simulink model "Control_v6_LQR_2020b_for_Monte_carlo"  (R2020b)
settings: Solver=FixedStepAuto  StartTime=0.0  StopTime=t_sim  FixedStep=TimeStep  RelTol=1e-3
values from neighbouring files (symbols this model uses):
  K = [mean(Kq1)  0  0  mean(Kw1)  0  0 ... (first row only)    [LQR_Compute_feedback_gain_matrix.m]    (also in LQR_Monte_Carlo_initial_conditions.m = [0.00053417  0  0  0.0070506  0  0; Main_LQR_Monte_Carlo_Simulations.m = [0.00053417  0  0  0.0070506  0  0)
  sat_inertia = [I_xx I_xy I_xz ... (first row only)    [Main_LQR_Monte_Carlo_Simulations.m]
  Use_IGRF = 1    [LQR_Monte_Carlo_initial_conditions.m]    (also in Main_LQR_Monte_Carlo_Simulations.m)
undefined symbols (not defined in the file or in its folder): att, date, deg, DiscIntNeverNeededParam, IonSataero, km, MODE_SEQUENCE, orbit, rad, RW_failure_matrix, s, sat
libraries: vrlib x23, aerolibutil x15, dspmathops x15, aerolibconvert2 x14, sharedtransform x13, simulink x4, simulink_extras x2, aerolibatmos2 x1, DipoleModel x1, aerolibobsolete x1, sharedutil x1, aerolibcelestial x1
(part 1 of 3)
settings Model: EnablePacing=on  PacingRate=1000  Creator=colpari  LastModifiedBy=shinok.kang
settings SolverCC: ExtrapolationOrder=3
settings OptimizationCC: DefaultParameterBehavior=Inlined  UseDivisionForNetSlopeComputation=on  GainParamInheritBuiltInType=on  UseFloatMulNetSlope=on  InlineInvariantSignals=on  EfficientFloat2IntCast=on  LifeSpan=1
settings HardwareCC: ProdLongLongMode=on
settings SFSimCC: MATLABDynamicMemAlloc=off
settings RTWCC: GenerateReport=on  LaunchReport=on
settings CodeAppCC: ForceParamTrailComments=on
settings GRTTargetCC: CombineSignalStateStructs=on  MatFileLogging=off  SupportVariableSizeSignals=on

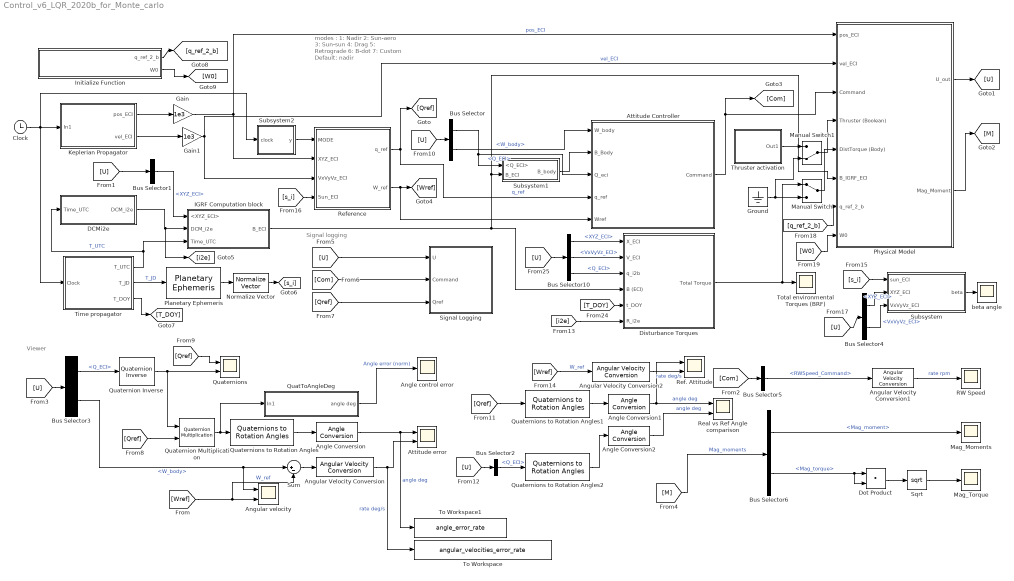
== system Control_v6_LQR_2020b_for_Monte_carlo ==
  note: Viewer
  note: Signal logging
  note: modes :
      | 1: Nadir
      | 2: Sun-aero
      | 3: Sun-sun
      | 4: Drag
      | 5: Retrograde
      | 6: B-dot
      | 7: Custom
      | Default: nadir
  Angle Conversion : aerolibconvert2/Angle Conversion  IU=rad  OU=deg
  Angle Conversion1 : aerolibconvert2/Angle Conversion  IU=rad  OU=deg
  Angle Conversion2 : aerolibconvert2/Angle Conversion  IU=rad  OU=deg
  Angle control error : Scope
  Angular Velocity Conversion : aerolibconvert2/Angular Velocity Conversion  IU=rad/s  OU=deg/s
  Angular Velocity Conversion1 : aerolibconvert2/Angular Velocity Conversion  IU=rad/s  OU=rpm
  Angular Velocity Conversion2 : aerolibconvert2/Angular Velocity Conversion  IU=rad/s  OU=deg/s
  Angular velocity : Scope  NumInputPorts=2
  Attitude Controller : Subsystem  TreatAsAtomicUnit=on
  Attitude error : Scope  NumInputPorts=2
  Bus Selector : BusSelector  OutputSignals=Q_ECI,W_body
  Bus Selector1 : BusSelector  OutputSignals=XYZ_ECI
  Bus Selector10 : BusSelector  OutputSignals=XYZ_ECI,VxVyVz_ECI,Q_ECI
  Bus Selector2 : BusSelector  OutputSignals=Q_ECI
  Bus Selector3 : BusSelector  OutputSignals=Q_ECI,W_body
  Bus Selector4 : BusSelector  OutputSignals=XYZ_ECI,VxVyVz_ECI
  Bus Selector5 : BusSelector  OutputSignals=RWSpeed_Command
  Bus Selector6 : BusSelector  OutputSignals=Mag_moment,Mag_torque
  Clock : Clock
  DCMi2e : Subsystem  TreatAsAtomicUnit=on  SystemSampleTime=1
  Disturbance Torques : Subsystem
  Dot Product : DotProduct  InputSameDT=on  OutDataTypeStr=Inherit: Inherit via internal rule
  Gain : Gain  Gain=1e3
  Gain1 : Gain  Gain=1e3
  Ground : Ground
  IGRF Computation block : Subsystem
  Initialize Function : Subsystem  TreatAsAtomicUnit=on
  Keplerian Propagator : Subsystem
  Mag_Moments : Scope
  Mag_Torque : Scope
  Manual Switch : ManualSwitch
  Manual Switch1 : ManualSwitch  CurrentSetting=0
  Normalize Vector : vrlib/Utilities/Normalize Vector  maxzero=0
  Physical Model : Subsystem
      settings: MinAlgLoopOccurrences=on
  Planetary Ephemeris : aerolibcelestial/Planetary Ephemeris  kmflag=km,km/s  epochflag=Julian date  de=DE405  nCenter=Earth  nTarget=Sun  errorflag=Error  velflag=off
      settings: SourceProductBaseCode=AE
  QuatToAngleDeg : Subsystem
  Quaternion Inverse : aerolibutil/Quaternion Inverse
  Quaternion Multiplication : aerolibutil/Quaternion Multiplication
  Quaternions : Scope  NumInputPorts=2
  Quaternions to Rotation Angles : sharedtransform/Quaternions to Rotation Angles  rotationOrder=ZYX  aMode=aMode
      settings: SourceProductBaseCode=AE,PW,DR,MT,UV,VE
  Quaternions to Rotation Angles1 : sharedtransform/Quaternions to Rotation Angles  rotationOrder=ZYX  aMode=aMode
      settings: SourceProductBaseCode=AE,PW,DR,MT,UV,VE
  Quaternions to Rotation Angles2 : sharedtransform/Quaternions to Rotation Angles  rotationOrder=ZYX  aMode=aMode
      settings: SourceProductBaseCode=AE,PW,DR,MT,UV,VE
  RW Speed : Scope
  Real vs Ref Angle comparison : Scope  NumInputPorts=2
  Ref. Attitude : Scope  NumInputPorts=2
  Reference : Subsystem  TreatAsAtomicUnit=on
  Signal Logging : Subsystem
  Sqrt : Sqrt  SaturateOnIntegerOverflow=on
  Subsystem : Subsystem
  Subsystem1 : Subsystem
  Subsystem2 : Subsystem
  Sum : Sum  Inputs=|+-
  Thruster activation : Subsystem
  Time propagator : Subsystem
  To Workspace : ToWorkspace  VariableName=angular_velocities_error_rate  SaveFormat=Timeseries  SampleTime=-1
  To Workspace1 : ToWorkspace  VariableName=angle_error_rate  SaveFormat=Timeseries  SampleTime=-1
  Total environmental Torques (BRF) : Scope
  beta angle : Scope
  wires:
  Clock/1 -> Subsystem2/1(clock), Keplerian Propagator/1(In1), Time propagator/1(Clock)
  Keplerian Propagator/1(pos_ECI) -> Gain/1
  Keplerian Propagator/2(vel_ECI) -> Gain1/1
  Planetary Ephemeris/1 -> Normalize Vector/1
  Time propagator/2(T_JD) -> Planetary Ephemeris/1  "T_JD"
  Reference/1(q_ref) -> [Qref], Attitude Controller/4(q_ref)  "q_ref"
  Physical Model/1(U_out) -> [U]
  Time propagator/1(T_UTC) -> DCMi2e/1(Time_UTC), IGRF Computation block/3("Time_UTC ")  "T_UTC"
  Gain/1 -> Reference/2(XYZ_ECI), Physical Model/1(pos_ECI)  "pos_ECI"
  Gain1/1 -> Reference/3(VxVyVz_ECI), Physical Model/2(vel_ECI)  "vel_ECI"
  Attitude Controller/1(Command) -> Physical Model/3(Command), [Com]
  IGRF Computation block/1(B_ECI) -> Physical Model/6(B_IGRF_ECI), Subsystem1/2(B_ECI), Disturbance Torques/4(B (ECI))
  [U] -> Bus Selector/1
  Bus Selector/1 -> Subsystem1/1(<Q_ECI>), Attitude Controller/3(Q_eci)  "<Q_ECI>"
  Bus Selector/2 -> Attitude Controller/1(W_body)  "<W_body>"
  [U] -> Bus Selector1/1
  Bus Selector1/1 -> IGRF Computation block/1(<XYZ_ECI>)  "<XYZ_ECI>"
  [Qref] -> Signal Logging/3(Qref)
  Quaternions to Rotation Angles/1 -> Angle Conversion/1
  Bus Selector6/2 -> Dot Product/2, Dot Product/1  "<Mag_torque>"
  Bus Selector6/1 -> Mag_Moments/1  "<Mag_moment>"
  Dot Product/1 -> Sqrt/1
  Bus Selector3/1 -> Quaternion Inverse/1  "<Q_ECI>"
  Sqrt/1 -> Mag_Torque/1
  Bus Selector5/1 -> Angular Velocity Conversion1/1  "<RWSpeed_Command>"
  [Com] -> Signal Logging/2(Command)
  [Com] -> Bus Selector5/1
  Bus Selector3/2 -> Sum/1, Angular velocity/1  "<W_body>"
  [U] -> Bus Selector3/1
  Quaternion Inverse/1 -> Quaternion Multiplication/1, Quaternions/2
  [M] -> Bus Selector6/1  "Mag_moments"
  Angular Velocity Conversion/1 -> To Workspace/1, Attitude error/2  "rate deg/s"
  Quaternion Multiplication/1 -> QuatToAngleDeg/1(In1), Quaternions to Rotation Angles/1
  [U] -> Signal Logging/1(U)
  Angle Conversion/1 -> To Workspace1/1, Attitude error/1  "angle deg"
  Angular Velocity Conversion1/1 -> RW Speed/1  "rate rpm"
  Physical Model/2(Mag_Moment) -> [M]
  Subsystem1/1(B_body) -> Attitude Controller/2(B_Body)
  QuatToAngleDeg/1(angle deg) -> Angle control error/1  "Angle error (norm)"
  Reference/2(W_ref) -> Attitude Controller/5(Wref), [Wref]
  [Wref] -> Sum/2, Angular velocity/2  "W_ref"
  Sum/1 -> Angular Velocity Conversion/1
  Angle Conversion1/1 -> Ref. Attitude/1, Real vs Ref Angle comparison/1  "angle deg"
  Quaternions to Rotation Angles1/1 -> Angle Conversion1/1
  Thruster activation/1(Out1) -> Manual Switch1/1
  [U] -> Bus Selector10/1
  [T_DOY] -> Disturbance Torques/5(t_DOY)
  Bus Selector10/3 -> Disturbance Torques/3(q_i2b)  "<Q_ECI>"
  Time propagator/3(T_DOY) -> [T_DOY]
  Manual Switch/1 -> Physical Model/5(DistTorque (Body))
  Ground/1 -> Manual Switch/2, Manual Switch1/2
  Bus Selector2/1 -> Quaternions to Rotation Angles2/1  "<Q_ECI>"
  Quaternions to Rotation Angles2/1 -> Angle Conversion2/1
  Angle Conversion2/1 -> Real vs Ref Angle comparison/2  "angle deg"
  [U] -> Bus Selector2/1
  [Wref] -> Angular Velocity Conversion2/1  "W_ref"
  Angular Velocity Conversion2/1 -> Ref. Attitude/2  "rate deg/s"
  DCMi2e/1(DCM_i2e) -> [i2e], IGRF Computation block/2("DCM_i2e ")
  [i2e] -> Disturbance Torques/6(R_i2e)
  Bus Selector10/1 -> Disturbance Torques/1(X_ECI)  "<XYZ_ECI>"
  Bus Selector10/2 -> Disturbance Torques/2(V_ECI)  "<VxVyVz_ECI>"
  Manual Switch1/1 -> Physical Model/4(Thruster (Boolean))
  Subsystem2/1(y) -> Reference/1(MODE)
  [s_i] -> Subsystem/1(sun_ECI)
  Subsystem/1(beta) -> beta angle/1
  Normalize Vector/1 -> [s_i]
  [s_i] -> Reference/4(Sun_ECI)
  [U] -> Bus Selector4/1
  Bus Selector4/1 -> Subsystem/2(XYZ_ECI)  "<XYZ_ECI>"
  Bus Selector4/2 -> Subsystem/3(VxVyVz_ECI)  "<VxVyVz_ECI>"
  Disturbance Torques/1("Total Torque ") -> Total environmental Torques (BRF)/1, Manual Switch/1
  [Qref] -> Quaternions to Rotation Angles1/1
  [Qref] -> Quaternions/1
  [Qref] -> Quaternion Multiplication/2
  Initialize Function/1(q_ref_2_b) -> [q_ref_2_b]
  [q_ref_2_b] -> Physical Model/7(q_ref_2_b)
  [W0] -> Physical Model/8(W0)
  Initialize Function/2(W0) -> [W0]

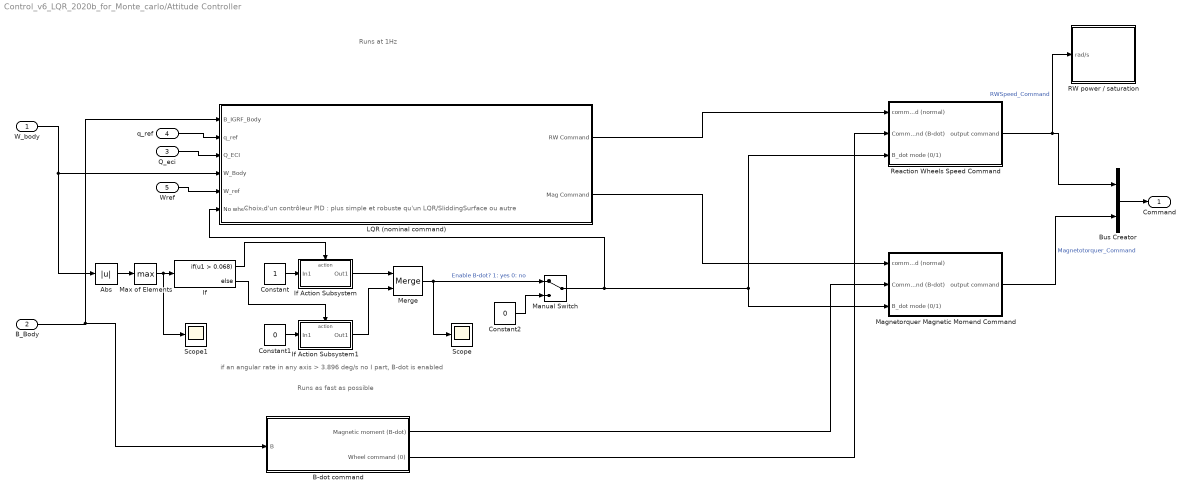
== system Control_v6_LQR_2020b_for_Monte_carlo/Attitude Controller ==
  note: Choix d'un contrôleur PID : plus simple et robuste qu'un LQR/SliddingSurface ou autre
  note: Runs as fast as possible
  note: Runs at 1Hz
  note: if an angular rate in any axis > 3.896 deg/s no I part, B-dot is enabled
  W_body : Inport
  B_Body : Inport  Port=2
  Q_eci : Inport  Port=3
  q_ref : Inport  Port=4
  Wref : Inport  Port=5
  Abs : Abs
  B-dot command : Subsystem  TreatAsAtomicUnit=on
  Bus Creator : BusCreator  Inputs=2
  Constant : Constant
  Constant1 : Constant  Value=0
  Constant2 : Constant  Value=0
  If : If  IfExpression=u1 > 0.068
  If Action Subsystem : Subsystem  TreatAsAtomicUnit=on
  If Action Subsystem1 : Subsystem  TreatAsAtomicUnit=on
  LQR (nominal command) : Subsystem  TreatAsAtomicUnit=on
  Magnetorquer Magnetic Momend Command : Subsystem
  Manual Switch : ManualSwitch
  Max of Elements : MinMax  Function=max
  Merge : Merge
  RW power / saturation : Subsystem
  Reaction Wheels Speed Command : Subsystem
  Scope : Scope
  Scope1 : Scope
  Command : Outport  VectorParamsAs1DForOutWhenUnconnected=off
  wires:
  B_Body/1 -> B-dot command/1(B), LQR (nominal command)/1(B_IGRF_Body)
  Magnetorquer Magnetic Momend Command/1(output command) -> Bus Creator/2  "Magnetotorquer_Command"
  Reaction Wheels Speed Command/1(output command) -> RW power / saturation/1(rad/s), Bus Creator/1  "RWSpeed_Command"
  B-dot command/2(Wheel command (0)) -> Reaction Wheels Speed Command/2(Command (B-dot))
  B-dot command/1(Magnetic moment (B-dot)) -> Magnetorquer Magnetic Momend Command/2(Command (B-dot))
  LQR (nominal command)/1(RW Command) -> Reaction Wheels Speed Command/1(" command (normal)")
  LQR (nominal command)/2(Mag Command) -> Magnetorquer Magnetic Momend Command/1(" command (normal)")
  Bus Creator/1 -> Command/1
  Abs/1 -> Max of Elements/1
  If/1 -> If Action Subsystem/Action
  If Action Subsystem1/1(Out1) -> Merge/2
  Max of Elements/1 -> Scope1/1, If/1
  If/2 -> If Action Subsystem1/Action
  If Action Subsystem/1(Out1) -> Merge/1
  Constant/1 -> If Action Subsystem/1(In1)
  Merge/1 -> Manual Switch/1, Scope/1  "Enable B-dot? 1: yes 0: no"
  Constant1/1 -> If Action Subsystem1/1(In1)
  W_body/1 -> Abs/1, LQR (nominal command)/4(W_Body)
  Wref/1 -> LQR (nominal command)/5(W_ref)
  q_ref/1 -> LQR (nominal command)/2(q_ref)
  Q_eci/1 -> LQR (nominal command)/3(Q_ECI)
  Constant2/1 -> Manual Switch/2
  Manual Switch/1 -> LQR (nominal command)/6(No wheels use), Reaction Wheels Speed Command/3(B_dot mode (0/1)), Magnetorquer Magnetic Momend Command/3(B_dot mode (0/1))

== system Control_v6_LQR_2020b_for_Monte_carlo/DCMi2e ==
  note: Slower subsytem because it's too slow
  Time_UTC : Inport
  ECI to ECEF : MATLABFcn  MATLABFcn=eci2ecef  OutputDimensions=[3;3]  Output1D=off
  DCM_i2e : Outport
  wires:
  ECI to ECEF/1 -> DCM_i2e/1
  Time_UTC/1 -> ECI to ECEF/1

== system Control_v6_LQR_2020b_for_Monte_carlo/Disturbance Torques ==
  X_ECI : Inport
  V_ECI : Inport  Port=2
  q_i2b : Inport  Port=3
  B (ECI) : Inport  Port=4
  t_DOY : Inport  Port=5
  R_i2e : Inport  Port=6
  3 dist torques : Scope  NumInputPorts=3
  Add1 : Sum  Inputs=+++
  Aerodynamic Model : Subsystem
  Gravity Gradient Model : Subsystem
  Ground : Ground
  Ground1 : Ground
  Ground2 : Ground
  Magnetic Torque Model : Subsystem
  Manual Switch : ManualSwitch
  Manual Switch1 : ManualSwitch
  Manual Switch2 : ManualSwitch
  Quaternions to Direction Cosine Matrix : sharedtransform/Quaternions to  Direction Cosine Matrix  aMode=aMode
      settings: SourceProductBaseCode=AE,PW,DR,MT,UV,VE
  To Workspace : ToWorkspace  VariableName=aerotorque  SaveFormat=Timeseries  SampleTime=-1
  Total Torque : Scope
  "Total Torque " : Outport
  wires:
  Add1/1 -> Total Torque/1, "Total Torque "/1
  V_ECI/1 -> Aerodynamic Model/1(Velocity  (V) [m/s])
  X_ECI/1 -> Aerodynamic Model/2(Position (X) [m]), Gravity Gradient Model/1("Position (X) [m] ")
  Manual Switch/1 -> 3 dist torques/1, Add1/1  "Aero Torque"
  Manual Switch2/1 -> Add1/3, 3 dist torques/3  "GG Torque"
  B (ECI)/1 -> Magnetic Torque Model/1(B (ECI))
  Manual Switch1/1 -> Add1/2, 3 dist torques/2  "Magnetic Torque"
  q_i2b/1 -> Quaternions to Direction Cosine Matrix/1
  Quaternions to Direction Cosine Matrix/1 -> Gravity Gradient Model/2(Attitude (DCMi2b)), Magnetic Torque Model/2(Attitude (DCMi2b)), Aerodynamic Model/3(Attitude (DCM_i2b))  "i2b"
  R_i2e/1 -> Aerodynamic Model/5(DCM_i2e)
  t_DOY/1 -> Aerodynamic Model/4(DOY)
  Ground/1 -> Manual Switch/2
  Aerodynamic Model/1(Aero. Torque [N.m]) -> To Workspace/1, Manual Switch/1  "Aero Torque"
  Magnetic Torque Model/1(MagneticTorque (N.m)) -> Manual Switch1/1  "Magnetic Torque"
  Ground1/1 -> Manual Switch1/2
  Ground2/1 -> Manual Switch2/2
  Gravity Gradient Model/1(Gravity Gradient [N.m]) -> Manual Switch2/1  "GG Torque"

== system Control_v6_LQR_2020b_for_Monte_carlo/IGRF Computation block ==
  <XYZ_ECI> : Inport
  "DCM_i2e " : Inport  Port=2
  "Time_UTC " : Inport  Port=3
  Bus Creator : BusCreator  Inputs=5
  Bus Selector4 : BusSelector  OutputSignals=XYZ_ECI
  Constant : Constant  Value=[0.4;0.4;0.4]
  Cross Product : vrlib/Utilities/Cross Product
  Demux : Demux  Outputs=2
  ECI To LLA : MATLAB Function  TreatAsAtomicUnit=on
  MATLAB Function : MATLAB Function  TreatAsAtomicUnit=on
  Mux : Mux  Inputs=3
  Obtain B_ECI : Subsystem
  Product : Product  Multiplication=Matrix(*)
  Reshape : Reshape  OutputDimensionality=Row vector (2-D)
  Scope : Scope
  Terminator : Terminator
  To Workspace : ToWorkspace  VariableName=B_ECI  SaveFormat=Timeseries  SampleTime=-1
  B_ECI : Outport  VectorParamsAs1DForOutWhenUnconnected=off
  wires:
  ECI To LLA/3(long) -> Bus Creator/3
  ECI To LLA/2(lat) -> Bus Creator/2
  ECI To LLA/1(h) -> Bus Creator/1
  Demux/1 -> Bus Creator/4  "time_UTC"
  Demux/2 -> Terminator/1
  "DCM_i2e "/1 -> Product/2, Bus Creator/5  "DCM_i2e"
  <XYZ_ECI>/1 -> Bus Selector4/1
  Reshape/1 -> Product/1
  Product/1 -> ECI To LLA/1(X_ECEF)
  Bus Selector4/1 -> Reshape/1  "<XYZ_ECI>"
  Bus Creator/1 -> Obtain B_ECI/1(In1)
  Obtain B_ECI/1(u) -> Cross Product/2, MATLAB Function/1(u), Mux/1, To Workspace/1, B_ECI/1
  "Time_UTC "/1 -> Demux/1
  Mux/1 -> Scope/1
  MATLAB Function/1(y) -> Mux/2
  Constant/1 -> Cross Product/1
  Cross Product/1 -> Mux/3

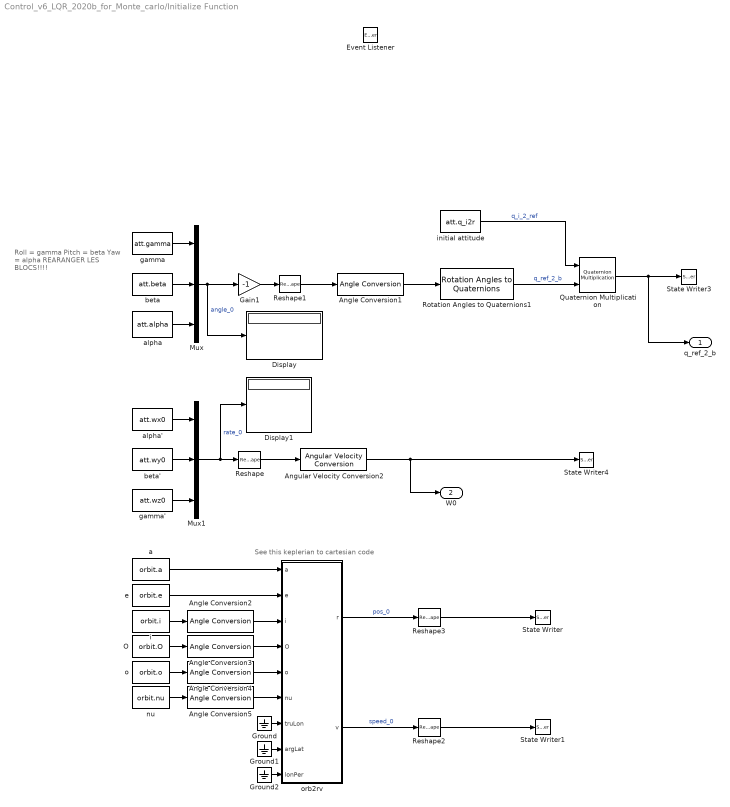
== system Control_v6_LQR_2020b_for_Monte_carlo/Initialize Function ==
  note: Roll = gamma
      | Pitch = beta
      | Yaw = alpha
      | REARANGER LES BLOCS!!!!
  note: See this keplerian to cartesian code
  Angle Conversion{1..5} (5 alike) : aerolibconvert2/Angle Conversion  IU=deg  OU=rad
  Angular Velocity Conversion2 : aerolibconvert2/Angular Velocity Conversion  IU=deg/s  OU=rad/s
  Display : Display
  Display1 : Display
  Event Listener : EventListener  DisableCoverage=on  EventName=reset
  Gain1 : Gain  Gain=-1
  Ground : Ground
  Ground1 : Ground
  Ground2 : Ground
  Mux : Mux  Inputs=3
  Mux1 : Mux  Inputs=3
  O : Constant  Value=orbit.O
  Quaternion Multiplication : aerolibutil/Quaternion Multiplication
  Reshape{,1..3} (4 alike) : Reshape  OutputDimensionality=Column vector (2-D)
  Rotation Angles to Quaternions1 : sharedtransform/Rotation Angles to Quaternions  rotationOrder=XYZ  aMode=aMode
      settings: SourceProductBaseCode=AE,PW,DR,MT,UV,VE
  State Writer : StateWriter  StateOwnerBlock=../../Keplerian Propagator/Integrator
  State Writer1 : StateWriter  StateOwnerBlock=../../Keplerian Propagator/Integrator1
  State Writer3 : StateWriter  StateOwnerBlock=../../Physical Model/6DOF in ECI frame/Compute Q_ECI/Integrator_quat
  State Writer4 : StateWriter  StateOwnerBlock=../../Physical Model/6DOF in ECI frame/Integrator_rate
  a : Constant  Value=orbit.a
  alpha : Constant  Value=att.alpha
  alpha' : Constant  Value=att.wx0
  beta : Constant  Value=att.beta
  beta' : Constant  Value=att.wy0
  e : Constant  Value=orbit.e
  gamma : Constant  Value=att.gamma
  gamma' : Constant  Value=att.wz0
  i : Constant  Value=orbit.i
  initial attitude : Constant  Value=att.q_i2r
  nu : Constant  Value=orbit.nu
  o : Constant  Value=orbit.o
  orb2rv : MATLAB Function  TreatAsAtomicUnit=on
  q_ref_2_b : Outport
  W0 : Outport  Port=2
  wires:
  Angular Velocity Conversion2/1 -> W0/1, State Writer4/1
  Mux1/1 -> Display1/1, Reshape/1  "rate_0"
  Reshape/1 -> Angular Velocity Conversion2/1
  alpha'/1 -> Mux1/1
  gamma'/1 -> Mux1/3
  beta'/1 -> Mux1/2
  Reshape3/1 -> State Writer/1
  i/1 -> Angle Conversion2/1
  Ground/1 -> orb2rv/7(truLon)
  Angle Conversion2/1 -> orb2rv/3(i)
  nu/1 -> Angle Conversion5/1
  Ground2/1 -> orb2rv/9(lonPer)
  Angle Conversion3/1 -> orb2rv/4(O)
  Angle Conversion5/1 -> orb2rv/6(nu)
  Ground1/1 -> orb2rv/8(argLat)
  o/1 -> Angle Conversion4/1
  a/1 -> orb2rv/1(a)
  O/1 -> Angle Conversion3/1
  orb2rv/2(v) -> Reshape2/1  "speed_0"
  e/1 -> orb2rv/2(e)
  orb2rv/1(r) -> Reshape3/1  "pos_0"
  Angle Conversion4/1 -> orb2rv/5(o)
  Reshape2/1 -> State Writer1/1
  Reshape1/1 -> Angle Conversion1/1
  Angle Conversion1/1 -> Rotation Angles to Quaternions1/1
  beta/1 -> Mux/2
  alpha/1 -> Mux/3
  gamma/1 -> Mux/1
  Mux/1 -> Gain1/1, Display/1  "angle_0"
  initial attitude/1 -> Quaternion Multiplication/1  "q_i_2_ref"
  Rotation Angles to Quaternions1/1 -> Quaternion Multiplication/2  "q_ref_2_b"
  Quaternion Multiplication/1 -> q_ref_2_b/1, State Writer3/1
  Gain1/1 -> Reshape1/1

== system Control_v6_LQR_2020b_for_Monte_carlo/Keplerian Propagator ==
  In1 : Inport
  Constant : Constant  Value=[0;0;0]
  Demux : Demux  Outputs=2
  Integrator : Integrator
  Integrator1 : Integrator
  Mux : Mux  Inputs=2
  Mux1 : Mux  Inputs=2
  Reshape1 : Reshape  OutputDimensionality=Customize  OutputDimensions=[6,1]
  Reshape3 : Reshape  OutputDimensionality=Column vector (2-D)
  keplerian propagator : MATLABFcn  MATLABFcn=kep_propagator
  pos_ECI : Outport
  vel_ECI : Outport  Port=2
  wires:
  Demux/2 -> vel_ECI/1  "vel_ECI"
  Demux/1 -> pos_ECI/1  "pos_ECI"
  keplerian propagator/1 -> Demux/1
  Mux1/1 -> keplerian propagator/1
  In1/1 -> Mux1/2
  Mux/1 -> Reshape1/1
  Reshape1/1 -> Mux1/1
  Integrator1/1 -> Mux/2
  Constant/1 -> Reshape3/1
  Reshape3/1 -> Integrator1/1, Integrator/1
  Integrator/1 -> Mux/1

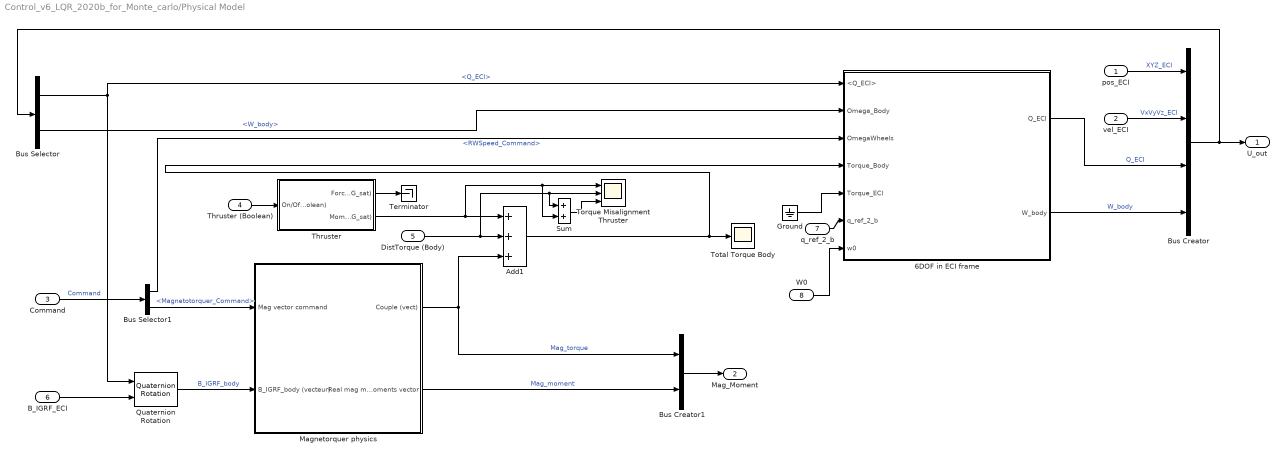
== system Control_v6_LQR_2020b_for_Monte_carlo/Physical Model ==
  pos_ECI : Inport
  vel_ECI : Inport  Port=2
  Command : Inport  Port=3
  Thruster (Boolean) : Inport  Port=4
  DistTorque (Body) : Inport  Port=5
  B_IGRF_ECI : Inport  Port=6
  q_ref_2_b : Inport  Port=7
  W0 : Inport  Port=8
  6DOF in ECI frame : Subsystem
  Add1 : Sum  Inputs=+++
  Bus Creator : BusCreator  Inputs=4
  Bus Creator1 : BusCreator  Inputs=2
  Bus Selector : BusSelector  OutputSignals=Q_ECI,W_body
  Bus Selector1 : BusSelector  OutputSignals=RWSpeed_Command,Magnetotorquer_Command
  Ground : Ground
  Magnetorquer physics : Subsystem
  Quaternion Rotation : aerolibutil/Quaternion Rotation
  Sum : Sum
  Terminator : Terminator
  Thruster : Subsystem
  Torque Misalignment Thruster : Scope  NumInputPorts=3
  Total Torque Body : Scope
  U_out : Outport  VectorParamsAs1DForOutWhenUnconnected=off
  Mag_Moment : Outport  Port=2  VectorParamsAs1DForOutWhenUnconnected=off
  wires:
  Thruster (Boolean)/1 -> Thruster/1(On/Off (Boolean))
  Bus Creator/1 -> U_out/1, Bus Selector/1
  Bus Selector/1 -> Quaternion Rotation/1, 6DOF in ECI frame/1(<Q_ECI>)  "<Q_ECI>"
  6DOF in ECI frame/1(Q_ECI) -> Bus Creator/3  "Q_ECI"
  Bus Selector1/2 -> Magnetorquer physics/1(Mag vector command)  "<Magnetotorquer_Command>"
  Thruster/2(Moment (G_sat)) -> Sum/2, Torque Misalignment Thruster/1, Add1/1
  Add1/1 -> Total Torque Body/1, 6DOF in ECI frame/4(Torque_Body)
  DistTorque (Body)/1 -> Sum/1, Torque Misalignment Thruster/2, Add1/2
  Bus Selector/2 -> 6DOF in ECI frame/2("Omega_Body ")  "<W_body>"
  B_IGRF_ECI/1 -> Quaternion Rotation/2
  Quaternion Rotation/1 -> Magnetorquer physics/2(B_IGRF_body (vecteur))  "B_IGRF_body"
  Magnetorquer physics/2(Real mag moments vector) -> Bus Creator1/2  "Mag_moment"
  Magnetorquer physics/1(Couple (vect)) -> Add1/3, Bus Creator1/1  "Mag_torque"
  6DOF in ECI frame/2(W_body) -> Bus Creator/4  "W_body"
  Command/1 -> Bus Selector1/1  "Command"
  Bus Selector1/1 -> 6DOF in ECI frame/3(OmegaWheels)  "<RWSpeed_Command>"
  Bus Creator1/1 -> Mag_Moment/1
  pos_ECI/1 -> Bus Creator/1  "XYZ_ECI"
  vel_ECI/1 -> Bus Creator/2  "VxVyVz_ECI"
  Thruster/1(Force (G_sat)) -> Terminator/1
  Ground/1 -> 6DOF in ECI frame/5(Torque_ECI)
  Sum/1 -> Torque Misalignment Thruster/3
  q_ref_2_b/1 -> 6DOF in ECI frame/6(q_ref_2_b)
  W0/1 -> 6DOF in ECI frame/7(w0)

== system Control_v6_LQR_2020b_for_Monte_carlo/QuatToAngleDeg ==
  In1 : Inport
  Abs : Abs
  Angle Conversion1 : aerolibconvert2/Angle Conversion  IU=rad  OU=deg
  Demux1 : Demux
  Quaternion to axis and angle conversion : MATLABFcn  MATLABFcn=quat2axisangle
  Terminator1 : Terminator
  Terminator2 : Terminator
  Terminator3 : Terminator
  angle deg : Outport  VectorParamsAs1DForOutWhenUnconnected=off
  wires:
  Demux1/2 -> Terminator2/1
  Demux1/4 -> Angle Conversion1/1
  In1/1 -> Quaternion to axis and angle conversion/1
  Demux1/1 -> Terminator1/1
  Demux1/3 -> Terminator3/1
  Quaternion to axis and angle conversion/1 -> Demux1/1
  Abs/1 -> angle deg/1
  Angle Conversion1/1 -> Abs/1  "angle deg"

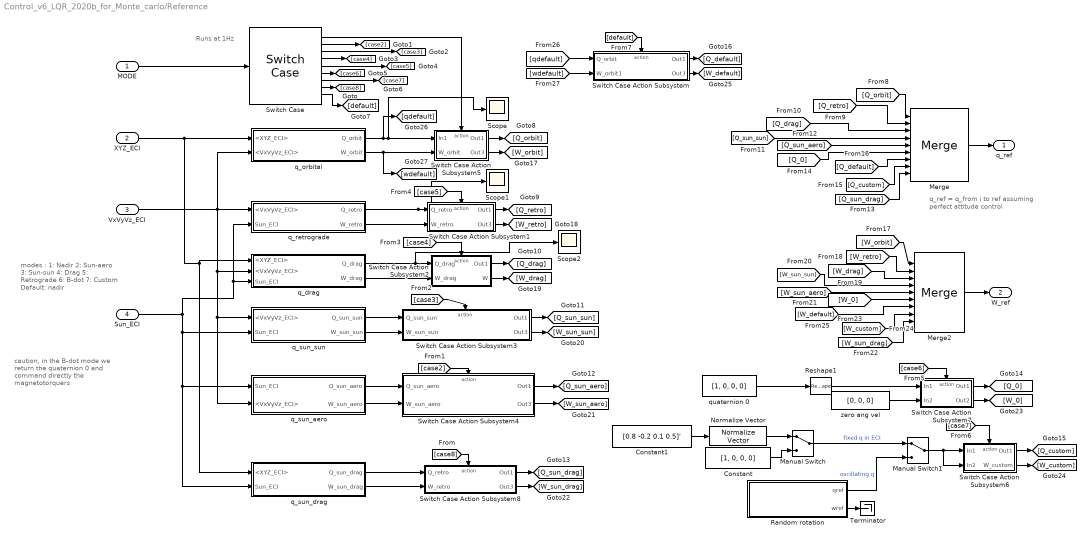
== system Control_v6_LQR_2020b_for_Monte_carlo/Reference ==
  note: caution, in the B-dot mode we return the quaternion 0 and command directly the magnetotorquers
  note: modes :
      | 1: Nadir
      | 2: Sun-aero
      | 3: Sun-sun
      | 4: Drag
      | 5: Retrograde
      | 6: B-dot
      | 7: Custom
      | Default: nadir
  note: q_ref  = q_from i to ref
      | assuming perfect attitude control
  note: Runs at 1Hz
  MODE : Inport  OutMin=1  OutMax=100  OutDataTypeStr=int8
  XYZ_ECI : Inport  Port=2
  VxVyVz_ECI : Inport  Port=3
  Sun_ECI : Inport  Port=4
  Constant : Constant  Value=[1, 0, 0, 0]
  Constant1 : Constant  Value=[0.8 -0.2 0.1 0.5]'
  Manual Switch : ManualSwitch
  Manual Switch1 : ManualSwitch
  Merge : Merge  Inputs=9
  Merge2 : Merge  Inputs=9
  Normalize Vector : vrlib/Utilities/Normalize Vector  maxzero=0
  Random rotation : Subsystem
  Reshape1 : Reshape  OutputDimensionality=Column vector (2-D)
  Scope : Scope
  Scope1 : Scope
  Scope2 : Scope
  Switch Case : SwitchCase  CaseConditions={1, 2, 3, 4, 5, 6, 7, 8}
  Switch Case Action Subsystem : Subsystem  TreatAsAtomicUnit=on
  Switch Case Action Subsystem1 : Subsystem  TreatAsAtomicUnit=on
  Switch Case Action Subsystem2 : Subsystem  TreatAsAtomicUnit=on
  Switch Case Action Subsystem3 : Subsystem  TreatAsAtomicUnit=on
  Switch Case Action Subsystem4 : Subsystem  TreatAsAtomicUnit=on
  Switch Case Action Subsystem5 : Subsystem  TreatAsAtomicUnit=on
  Switch Case Action Subsystem6 : Subsystem  TreatAsAtomicUnit=on
  Switch Case Action Subsystem7 : Subsystem  TreatAsAtomicUnit=on
  Switch Case Action Subsystem8 : Subsystem  TreatAsAtomicUnit=on
  Terminator : Terminator
  q_drag : Subsystem
  q_orbital : Subsystem
  q_retrograde : Subsystem
  q_sun_aero : Subsystem
  q_sun_drag : Subsystem
  q_sun_sun : Subsystem
  quaternion 0 : Constant  Value=[1, 0, 0, 0]
  zero ang vel : Constant  Value=[0, 0, 0]
  q_ref : Outport  VectorParamsAs1DForOutWhenUnconnected=off
  W_ref : Outport  Port=2
  wires:
  quaternion 0/1 -> Reshape1/1
  Reshape1/1 -> Switch Case Action Subsystem7/1(In1)
  Constant/1 -> Manual Switch/2
  Constant1/1 -> Normalize Vector/1
  Normalize Vector/1 -> Manual Switch/1
  zero ang vel/1 -> Switch Case Action Subsystem7/2(In2)
  Manual Switch/1 -> Manual Switch1/1  "fixed q in ECI"
  Random rotation/1(qref) -> Manual Switch1/2  "oscillating q"
  Manual Switch1/1 -> Switch Case Action Subsystem6/2(In2), Switch Case Action Subsystem6/1(In1)
  XYZ_ECI/1 -> q_sun_drag/1(<XYZ_ECI>), q_drag/1(<XYZ_ECI>), q_orbital/1(<XYZ_ECI>)
  [default] -> Switch Case Action Subsystem/Action
  Switch Case/7 -> [case7]
  Switch Case/4 -> [case4]
  Switch Case/5 -> [case5]
  [case3] -> Switch Case Action Subsystem3/Action
  [case5] -> Switch Case Action Subsystem1/Action
  Switch Case/3 -> [case3]
  Switch Case/2 -> [case2]
  q_drag/2(W_drag) -> Switch Case Action Subsystem2/2(W_drag)
  q_sun_drag/2(W_sun_drag) -> Switch Case Action Subsystem8/2(W_retro)
  q_sun_aero/2(W_sun_aero) -> Switch Case Action Subsystem4/2(W_sun_aero)
  Switch Case/1 -> Switch Case Action Subsystem5/Action
  [case8] -> Switch Case Action Subsystem8/Action
  Switch Case/8 -> [case8]
  q_drag/1(Q_drag) -> Scope2/1, Switch Case Action Subsystem2/1(Q_drag)
  Switch Case/9 -> [default]
  Sun_ECI/1 -> q_drag/3(Sun_ECI), q_retrograde/2(Sun_ECI), q_sun_drag/2(Sun_ECI), q_sun_aero/1(Sun_ECI), q_sun_sun/2(Sun_ECI)
  q_sun_sun/2(W_sun_sun) -> Switch Case Action Subsystem3/2(W_sun_sun)
  q_retrograde/2(W_retro) -> Switch Case Action Subsystem1/2(W_retro)
  q_sun_sun/1(Q_sun_sun) -> Switch Case Action Subsystem3/1(Q_sun_sun)
  q_sun_aero/1(Q_sun_aero) -> Switch Case Action Subsystem4/1(Q_sun_aero)
  q_sun_drag/1(Q_sun_drag) -> Switch Case Action Subsystem8/1(Q_retro)
  Merge2/1 -> W_ref/1
  [case2] -> Switch Case Action Subsystem4/Action
  [case4] -> Switch Case Action Subsystem2/Action
  q_orbital/1(Q_orbit) -> [qdefault], Switch Case Action Subsystem5/1(In1), Scope/1
  q_retrograde/1(Q_retro) -> Switch Case Action Subsystem1/1(Q_retro), Scope1/1
  q_orbital/2(W_orbit) -> [wdefault], Switch Case Action Subsystem5/2(W_orbit)
  Switch Case/6 -> [case6]
  VxVyVz_ECI/1 -> q_orbital/2(<VxVyVz_ECI>), q_retrograde/1(<VxVyVz_ECI>), q_sun_aero/2(<VxVyVz_ECI>), q_sun_sun/1(<VxVyVz_ECI>), q_drag/2(<VxVyVz_ECI>)
  Merge/1 -> q_ref/1
  MODE/1 -> Switch Case/1
  Random rotation/2(wref) -> Terminator/1
  [case6] -> Switch Case Action Subsystem7/Action
  [case7] -> Switch Case Action Subsystem6/Action
  Switch Case Action Subsystem5/1(Out1) -> [Q_orbit]
  [Q_orbit] -> Merge/1
  Switch Case Action Subsystem1/1(Out1) -> [Q_retro]
  [Q_retro] -> Merge/2
  Switch Case Action Subsystem2/1(Out1) -> [Q_drag]
  [Q_drag] -> Merge/3
  Switch Case Action Subsystem3/1(Out1) -> [Q_sun_sun]
  [Q_sun_sun] -> Merge/4
  Switch Case Action Subsystem4/1(Out1) -> [Q_sun_aero]
  [Q_sun_aero] -> Merge/5
  Switch Case Action Subsystem8/1(Out1) -> [Q_sun_drag]
  [Q_sun_drag] -> Merge/9
  Switch Case Action Subsystem7/1(Out1) -> [Q_0]
  [Q_0] -> Merge/6
  Switch Case Action Subsystem6/1(Out1) -> [Q_custom]
  [Q_custom] -> Merge/8
  Switch Case Action Subsystem/1(Out1) -> [Q_default]
  [Q_default] -> Merge/7
  Switch Case Action Subsystem5/2(Out3) -> [W_orbit]
  [W_orbit] -> Merge2/1
  Switch Case Action Subsystem1/2(Out3) -> [W_retro]
  [W_retro] -> Merge2/2
  Switch Case Action Subsystem2/2(W) -> [W_drag]
  [W_drag] -> Merge2/3
  Switch Case Action Subsystem3/2(Out3) -> [W_sun_sun]
  [W_sun_sun] -> Merge2/4
  Switch Case Action Subsystem4/2(Out3) -> [W_sun_aero]
  [W_sun_aero] -> Merge2/5
  Switch Case Action Subsystem8/2(Out3) -> [W_sun_drag]
  [W_sun_drag] -> Merge2/9
  Switch Case Action Subsystem7/2(Out2) -> [W_0]
  [W_0] -> Merge2/6
  Switch Case Action Subsystem6/2(W_custom) -> [W_custom]
  [W_custom] -> Merge2/8
  Switch Case Action Subsystem/2(Out3) -> [W_default]
  [W_default] -> Merge2/7
  [qdefault] -> Switch Case Action Subsystem/1(Q_orbit)
  [wdefault] -> Switch Case Action Subsystem/2(W_orbit1)

== system Control_v6_LQR_2020b_for_Monte_carlo/Signal Logging ==
  U : Inport
  Command : Inport  Port=2
  Qref : Inport  Port=3
  Bus Selector : BusSelector  OutputSignals=RWSpeed_Command,Magnetotorquer_Command
  Bus Selector4 : BusSelector  OutputSignals=XYZ_ECI,VxVyVz_ECI,Q_ECI,W_body
  Reshape : Reshape
  Reshape1 : Reshape
  Reshape2 : Reshape
  To Workspace : ToWorkspace  VariableName=sat_pos  SaveFormat=Timeseries  SampleTime=1
      settings: Save2DSignal=2-D array (concatenate along first dimension)
  To Workspace1 : ToWorkspace  VariableName=sat_speed  SaveFormat=Timeseries  SampleTime=1
      settings: Save2DSignal=2-D array (concatenate along first dimension)
  To Workspace2 : ToWorkspace  VariableName=sat_Q  SaveFormat=Timeseries  SampleTime=1
      settings: Save2DSignal=2-D array (concatenate along first dimension)
  To Workspace3 : ToWorkspace  VariableName=sat_omega  SaveFormat=Timeseries  SampleTime=1
      settings: Save2DSignal=2-D array (concatenate along first dimension)
  To Workspace4 : ToWorkspace  VariableName=RWSpeed_Command  SaveFormat=Timeseries  SampleTime=1
      settings: Save2DSignal=2-D array (concatenate along first dimension)
  To Workspace5 : ToWorkspace  VariableName=sat_Qc  SaveFormat=Timeseries  SampleTime=1
      settings: Save2DSignal=2-D array (concatenate along first dimension)
  To Workspace6 : ToWorkspace  VariableName=Mag_Command  SaveFormat=Timeseries  SampleTime=1
      settings: Save2DSignal=2-D array (concatenate along first dimension)
  wires:
  Bus Selector4/3 -> To Workspace2/1  "<Q_ECI>"
  Bus Selector4/4 -> To Workspace3/1  "<W_body>"
  U/1 -> Bus Selector4/1
  Bus Selector4/2 -> To Workspace1/1  "<VxVyVz_ECI>"
  Command/1 -> Bus Selector/1
  Bus Selector4/1 -> To Workspace/1  "<XYZ_ECI>"
  Qref/1 -> Reshape1/1
  Reshape/1 -> To Workspace4/1
  Reshape1/1 -> To Workspace5/1
  Bus Selector/1 -> Reshape/1  "<RWSpeed_Command>"
  Bus Selector/2 -> Reshape2/1  "<Magnetotorquer_Command>"
  Reshape2/1 -> To Workspace6/1

== system Control_v6_LQR_2020b_for_Monte_carlo/Subsystem ==
  sun_ECI : Inport
  XYZ_ECI : Inport  Port=2
  VxVyVz_ECI : Inport  Port=3
  Acos : Trigonometry  Operator=acos
  Constant1 : Constant  Value=90
  Cross Product : vrlib/Utilities/Cross Product
  Dot Product1 : DotProduct  InputSameDT=on  OutDataTypeStr=Inherit: Inherit via internal rule
  Gain2 : Gain  Gain=180/pi
  Normalize Vector2 : vrlib/Utilities/Normalize Vector  maxzero=0
  Sum1 : Sum  Inputs=|-+
  beta : Outport
  wires:
  Constant1/1 -> Sum1/2
  Acos/1 -> Gain2/1
  Dot Product1/1 -> Acos/1
  Cross Product/1 -> Normalize Vector2/1
  Gain2/1 -> Sum1/1
  VxVyVz_ECI/1 -> Cross Product/2
  XYZ_ECI/1 -> Cross Product/1  "pos_ECI"
  Normalize Vector2/1 -> Dot Product1/2  "x"
  sun_ECI/1 -> Dot Product1/1
  Sum1/1 -> beta/1

== system Control_v6_LQR_2020b_for_Monte_carlo/Subsystem1 ==
  <Q_ECI> : Inport
  B_ECI : Inport  Port=2
  Quaternion Rotation : aerolibutil/Quaternion Rotation
  B_body : Outport
  wires:
  <Q_ECI>/1 -> Quaternion Rotation/1
  B_ECI/1 -> Quaternion Rotation/2
  Quaternion Rotation/1 -> B_body/1  "B_IGRF_body"

== system Control_v6_LQR_2020b_for_Monte_carlo/Subsystem2 ==
  clock : Inport
  MATLAB Function : MATLAB Function  TreatAsAtomicUnit=on
  Mode : Constant  Value=MODE_SEQUENCE  OutDataTypeStr=int8
  Scope : Scope
  y : Outport
  wires:
  Mode/1 -> MATLAB Function/1(mode_sequence)
  MATLAB Function/1(actual_mode) -> Scope/1, y/1
  clock/1 -> MATLAB Function/2(clock)

== system Control_v6_LQR_2020b_for_Monte_carlo/Thruster activation ==
  Clock1 : Clock
  Constant3 : Constant  Value=sat.thruster.duration
  Constant4 : Constant  Value=sat.thruster.firstimpulse
  Constant5 : Constant  Value=sat.thruster.wait
  Constant6 : Constant  Value=sat.thruster.Nfirings
  MATLAB Function : MATLAB Function  TreatAsAtomicUnit=on
  Mux1 : Mux  Inputs=5
  Scope : Scope
  Out1 : Outport  VectorParamsAs1DForOutWhenUnconnected=off
  wires:
  MATLAB Function/1(y) -> Scope/1, Out1/1
  Clock1/1 -> Mux1/1
  Constant4/1 -> Mux1/3
  Constant6/1 -> Mux1/5
  Mux1/1 -> MATLAB Function/1(u)
  Constant3/1 -> Mux1/2
  Constant5/1 -> Mux1/4

== system Control_v6_LQR_2020b_for_Monte_carlo/Time propagator ==
  note: Time initialization
  Clock : Inport
  Add : Sum  Inputs=|++
  Constant : Constant  Value=86400
  Day : Constant  Value=date.day
  Divide : Product  Inputs=*/
  HH : Constant  Value=date.hours
  JD to UTC : MATLAB Function  TreatAsAtomicUnit=on
  MATLAB Function : MATLAB Function  TreatAsAtomicUnit=on
  MM : Constant  Value=date.minutes
  Month : Constant  Value=date.month
  Mux : Mux  Inputs=6
  Mux1 : Mux  Inputs=3
  Reshape : Reshape
  SS : Constant  Value=date.seconds
  Signal logging : ToWorkspace  VariableName=T_UTC  SaveFormat=Timeseries  SampleTime=1
      settings: Save2DSignal=2-D array (concatenate along first dimension)
  Signal logging1 : ToWorkspace  VariableName=T_JD  SaveFormat=Timeseries  SampleTime=1
      settings: Save2DSignal=2-D array (concatenate along first dimension)
  UTC to JD : MATLAB Function  TreatAsAtomicUnit=on
  Year : Constant  Value=date.year
  T_UTC : Outport  VectorParamsAs1DForOutWhenUnconnected=off
  T_JD : Outport  Port=2  VectorParamsAs1DForOutWhenUnconnected=off
  T_DOY : Outport  Port=3
  wires:
  UTC to JD/1(JD) -> Add/1  "JD_0"
  Constant/1 -> Divide/2
  JD to UTC/1(Time_UTC) -> T_UTC/1, Reshape/1
  Divide/1 -> Add/2
  Mux/1 -> UTC to JD/1(Time_UTC)
  Day/1 -> Mux/3
  Month/1 -> Mux/2
  Year/1 -> Mux/1
  HH/1 -> Mux/4
  MM/1 -> Mux/5
  SS/1 -> Mux/6
  Reshape/1 -> Signal logging/1
  Add/1 -> Signal logging1/1, T_JD/1, JD to UTC/1(JD)
  MATLAB Function/1(Y) -> Mux1/1
  MATLAB Function/2(DOY) -> Mux1/2
  MATLAB Function/3(S) -> Mux1/3
  Mux1/1 -> T_DOY/1
  Clock/1 -> MATLAB Function/1(t), Divide/1

== system Control_v6_LQR_2020b_for_Monte_carlo/Attitude Controller/B-dot command ==
  note: ref : OneDrive\IonSat X18\SCAO\Contrôle attitude\Detumbling\Detumbling and Aerostable Control for Cubesats.pdf
      |
      | formulae:
      | $\mathbf{\dot B} \simeq \mathbf{B}\times \mathbf{\dot \theta}$
      | $\mathbf{m} = -c\mathbf{\dot B}$
      |
      | this block does NOT decide if the B-dot mode is relevant or not
      | (it applies it without question on the rotation rate :
      | $\Omega=v/r= \sqrt{\frac{Gm_{earth}}{(h+r_{earth})^{3/2}}} \sim 0.066 °/s$ So the command MUST stop the B-dot mode when the estimated rotation speed is smaller than 0.1 degree per second )
  note: entrée:
      | champ magnétique
      | sortie: moment magnetique de commande et vitesse des roues à réaction (nulle)
  B : Inport
  Discrete Derivative : simulink/Discrete/Discrete Derivative  gainval=1.0  ICPrevScaledInput=0.0  OutMin=[]  OutMax=[]  OutDataType=fixdt(1, 16)  OutScaling=2^-10  DoSatur=off
  Divide1 : Product  Inputs=**
  Reshape2 : Reshape  OutputDimensionality=Column vector (2-D)
  constant c : Constant  Value=-sat.bdot_c
  wheels unused : Constant  Value=[0, 0, 0, 0]
  Magnetic moment (B-dot) : Outport  VectorParamsAs1DForOutWhenUnconnected=off
  Wheel command (0) : Outport  Port=2  VectorParamsAs1DForOutWhenUnconnected=off
  wires:
  constant c/1 -> Divide1/2
  B/1 -> Discrete Derivative/1
  Discrete Derivative/1 -> Divide1/1  "B_point=B^theta_point"
  Divide1/1 -> Magnetic moment (B-dot)/1
  wheels unused/1 -> Reshape2/1
  Reshape2/1 -> Wheel command (0)/1

== system Control_v6_LQR_2020b_for_Monte_carlo/Attitude Controller/If Action Subsystem ==
  In1 : Inport
  Action Port : ActionPort  ActionPortLabel=if(u1 > 0.068)
  Out1 : Outport  VectorParamsAs1DForOutWhenUnconnected=off
  wires:
  In1/1 -> Out1/1

== system Control_v6_LQR_2020b_for_Monte_carlo/Attitude Controller/If Action Subsystem1 ==
  In1 : Inport
  Action Port : ActionPort  ActionPortLabel=else
  Out1 : Outport  VectorParamsAs1DForOutWhenUnconnected=off
  wires:
  In1/1 -> Out1/1

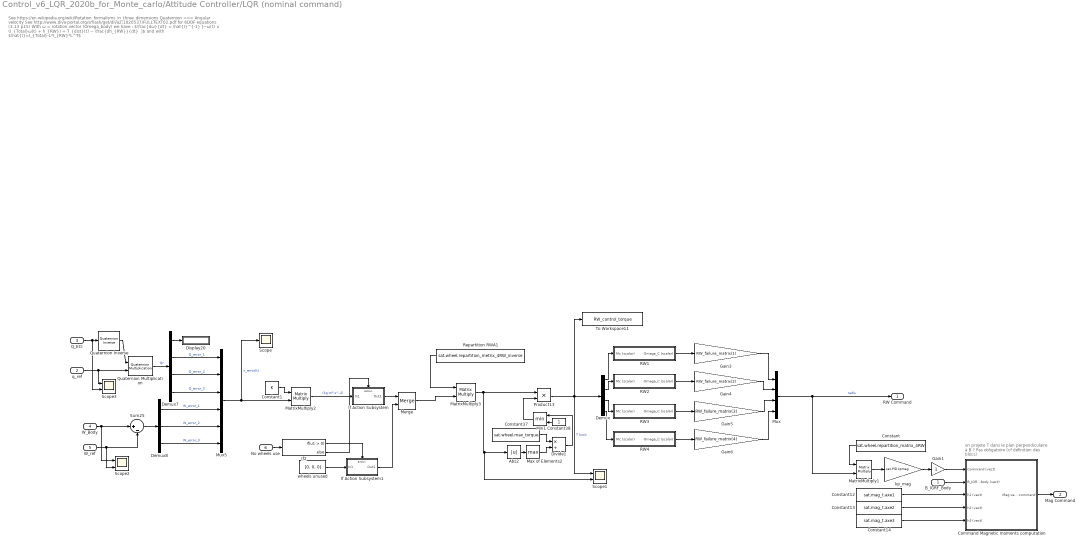
== system Control_v6_LQR_2020b_for_Monte_carlo/Attitude Controller/LQR (nominal command) ==
  note: on projete T dans
      | le plan perpendiculaire à B ?
      | Pas obligatoire (cf définition des blocs)
  note: See https://en.wikipedia.org/wiki/Rotation_formalisms_in_three_dimensions Quaternion <=> Angular velocity
      |
      | See http://www.diva-portal.org/smash/get/diva2:1020537/FULLTEXT02.pdf for 6DOF equations (3.13 p15)
      |
      | With ω = rotation vector (Omega_body) we have :
      |
      | $\frac{dω}{dt} = \hat{I}^{-1} [−ω(t) × (I_{Total}ω(t) + h_{RW}) + T_{dist}(t) − \frac{dh_{RW}}{dt} ̇ ]$
      | and with $\hat{I}=I_{Total}-L*I_{RW}*L^T$
  B_IGRF_Body : Inport
  q_ref : Inport  Port=2
  Q_ECI : Inport  Port=3
  W_Body : Inport  Port=4
  W_ref : Inport  Port=5
  No wheels use : Inport  Port=6
  Abs2 : Abs
  Command Magnetic moments computation : Subsystem
  Constant : Constant  Value=sat.wheel.repartition_matrix_4RW
  Constant1 : Constant  Value=K
  Constant12 : Constant  Value=sat.mag_t.axe1
  Constant13 : Constant  Value=sat.mag_t.axe2
  Constant14 : Constant  Value=sat.mag_t.axe3
  Constant37 : Constant  Value=sat.wheel.max_torque
  Constant38 : Constant
  Demux : Demux
  Demux7 : Demux
  Demux8 : Demux  Outputs=3
  Display20 : Display
  Divide1 : Product  Inputs=*/
  Gain1 : Gain
  Gain3 : Gain  Gain=RW_failure_matrix(1)
  Gain4 : Gain  Gain=RW_failure_matrix(2)
  Gain5 : Gain  Gain=RW_failure_matrix(3)
  Gain6 : Gain  Gain=RW_failure_matrix(4)
  If Action Subsystem : Subsystem  TreatAsAtomicUnit=on
  If Action Subsystem1 : Subsystem  TreatAsAtomicUnit=on
  If2 : If
  MatrixMultiply1 : Product  Multiplication=Matrix(*)
  MatrixMultiply2 : Product  Multiplication=Matrix(*)
  MatrixMultiply3 : Product  Multiplication=Matrix(*)
  Max of Elements2 : MinMax  Function=max
  Merge : Merge
  Min1 : MinMax  Inputs=2
  Mux : Mux
  Mux5 : Mux  Inputs=6
  Product13 : Product
  Quaternion Inverse : aerolibutil/Quaternion Inverse
  Quaternion Multiplication : aerolibutil/Quaternion Multiplication
  RW1 : Subsystem
  RW2 : Subsystem
  RW3 : Subsystem
  "RW4 " : Subsystem
  Repartition RWA1 : Constant  Value=sat.wheel.repartition_metrix_4RW_inverse
  Scope : Scope
  Scope1 : Scope  NumInputPorts=2
  Scope2 : Scope  NumInputPorts=2
  Scope3 : Scope  NumInputPorts=2
  Sum25 : Sum  Inputs=|+-
  To Workspace11 : ToWorkspace  VariableName=RW_control_torque  SaveFormat=Timeseries  SampleTime=-1
  kp_mag : Gain  Gain=sat.PID.kpmag
  wheels unused : Constant  Value=[0, 0, 0]
  RW Command : Outport  VectorParamsAs1DForOutWhenUnconnected=off
  Mag Command : Outport  Port=2  VectorParamsAs1DForOutWhenUnconnected=off
  wires:
  Command Magnetic moments computation/1(Mag vector command) -> Mag Command/1
  Constant14/1 -> Command Magnetic moments computation/5(h3 (vect))
  Constant12/1 -> Command Magnetic moments computation/3(h1 (vect))
  Constant/1 -> MatrixMultiply1/1
  Demux/4 -> "RW4 "/1(Mc (scalar))
  Constant13/1 -> Command Magnetic moments computation/4(h2 (vect))
  Demux/3 -> RW3/1(Mc (scalar))
  RW3/1(Omega_C (scalar)) -> Gain5/1
  RW2/1(Omega_C (scalar)) -> Gain4/1
  Demux/2 -> RW2/1(Mc (scalar))
  Demux/1 -> RW1/1(Mc (scalar))
  Gain1/1 -> Command Magnetic moments computation/1(Command (vect))
  B_IGRF_Body/1 -> Command Magnetic moments computation/2(B_IGRF_body (vect))
  "RW4 "/1(Omega_C (scalar)) -> Gain6/1
  kp_mag/1 -> Gain1/1
  MatrixMultiply1/1 -> kp_mag/1
  RW1/1(Omega_C (scalar)) -> Gain3/1
  Mux/1 -> MatrixMultiply1/2, RW Command/1  "rad/s"
  q_ref/1 -> Scope3/1, Quaternion Multiplication/2
  Quaternion Inverse/1 -> Quaternion Multiplication/1
  Q_ECI/1 -> Scope3/2, Quaternion Inverse/1
  W_ref/1 -> Scope2/2, Sum25/2
  W_Body/1 -> Sum25/1, Scope2/1
  Quaternion Multiplication/1 -> Demux7/1  "Qr"
  Demux8/3 -> Mux5/6  "W_error_3"
  Demux8/1 -> Mux5/4  "W_error_1"
  Demux7/2 -> Mux5/1  "Q_error_1"
  Demux8/2 -> Mux5/5  "W_error_2"
  Demux7/4 -> Mux5/3  "Q_error_3"
  Demux7/3 -> Mux5/2  "Q_error_2"
  Sum25/1 -> Demux8/1
  Demux7/1 -> Display20/1
  Mux5/1 -> MatrixMultiply2/2, Scope/1  "x_error(t)"
  Repartition RWA1/1 -> MatrixMultiply3/1
  MatrixMultiply2/1 -> If Action Subsystem/1(In1)  "(kg.m².s^-2)"
  Abs2/1 -> Max of Elements2/1
  Constant37/1 -> Divide1/1
  Min1/1 -> Product13/2
  Divide1/1 -> Min1/1
  Constant38/1 -> Min1/2
  Max of Elements2/1 -> Divide1/2
  Product13/1 -> Scope1/1, Demux/1, To Workspace11/1  "T limit"
  MatrixMultiply3/1 -> Scope1/2, Abs2/1, Product13/1
  Constant1/1 -> MatrixMultiply2/1
  If2/1 -> If Action Subsystem1/Action
  wheels unused/1 -> If Action Subsystem1/1(In1)
  No wheels use/1 -> If2/1
  If Action Subsystem/1(Out1) -> Merge/1
  Merge/1 -> MatrixMultiply3/2
  If2/2 -> If Action Subsystem/Action
  If Action Subsystem1/1(Out1) -> Merge/2
  Gain3/1 -> Mux/1
  Gain4/1 -> Mux/2
  Gain5/1 -> Mux/3
  Gain6/1 -> Mux/4

== system Control_v6_LQR_2020b_for_Monte_carlo/Attitude Controller/Magnetorquer Magnetic Momend Command ==
  " command (normal)" : Inport
  Command (B-dot) : Inport  Port=2
  B_dot mode (0/1) : Inport  Port=3
  If1 : If
  Merge : Merge
  Switch Case Action Subsystem3 : Subsystem  TreatAsAtomicUnit=on
  Switch Case Action Subsystem4 : Subsystem  TreatAsAtomicUnit=on
  output command : Outport  VectorParamsAs1DForOutWhenUnconnected=off
  wires:
  If1/2 -> Switch Case Action Subsystem4/Action
  If1/1 -> Switch Case Action Subsystem3/Action
  B_dot mode (0/1)/1 -> If1/1
  Command (B-dot)/1 -> Switch Case Action Subsystem3/1(In1)
  Switch Case Action Subsystem3/1(Out1) -> Merge/1
  Switch Case Action Subsystem4/1(Out1) -> Merge/2
  " command (normal)"/1 -> Switch Case Action Subsystem4/1(In1)
  Merge/1 -> output command/1

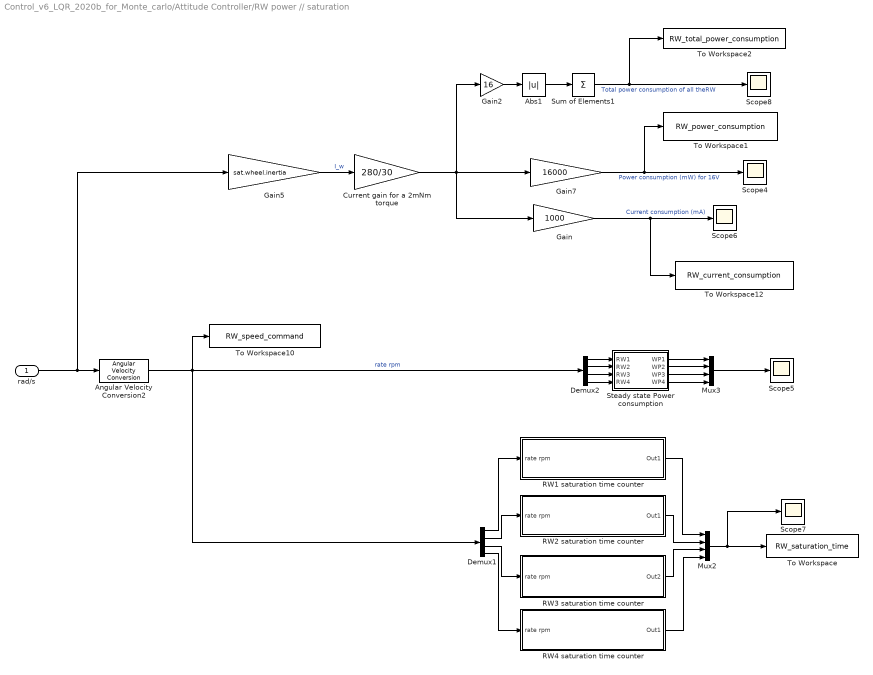
== system Control_v6_LQR_2020b_for_Monte_carlo/Attitude Controller/RW power // saturation ==
  rad/s : Inport
  Abs1 : Abs
  Angular Velocity Conversion2 : aerolibconvert2/Angular Velocity Conversion  IU=rad/s  OU=rpm
  Current gain for a 2mNm torque : Gain  Gain=280/30
  Demux1 : Demux
  Demux2 : Demux
  Gain : Gain  Gain=1000
  Gain2 : Gain  Gain=16
  Gain5 : Gain  Gain=sat.wheel.inertia
  Gain7 : Gain  Gain=16000
  Mux2 : Mux
  Mux3 : Mux
  RW1 saturation time counter : Subsystem
  RW2 saturation time counter : Subsystem
  RW3 saturation time counter : Subsystem
  RW4 saturation time counter : Subsystem
  Scope{4..8} (5 alike) : Scope
  Steady state Power consumption : MATLAB Function  TreatAsAtomicUnit=on
  Sum of Elements1 : Sum  Inputs=+
  To Workspace : ToWorkspace  VariableName=RW_saturation_time  SaveFormat=Timeseries  SampleTime=-1
  To Workspace1 : ToWorkspace  VariableName=RW_power_consumption  SaveFormat=Timeseries  SampleTime=-1
  To Workspace10 : ToWorkspace  VariableName=RW_speed_command  SaveFormat=Timeseries  SampleTime=-1
  To Workspace12 : ToWorkspace  VariableName=RW_current_consumption  SaveFormat=Timeseries  SampleTime=-1
  To Workspace2 : ToWorkspace  VariableName=RW_total_power_consumption  SaveFormat=Timeseries  SampleTime=-1
  wires:
  Demux1/3 -> RW3 saturation time counter/1(rate rpm)
  RW2 saturation time counter/1(Out1) -> Mux2/2
  Abs1/1 -> Sum of Elements1/1
  Gain7/1 -> To Workspace1/1, Scope4/1  "Power consumption (mW) for 16V"
  Demux1/4 -> RW4 saturation time counter/1(rate rpm)
  Demux2/2 -> Steady state Power consumption/2(RW2)
  Mux2/1 -> Scope7/1, To Workspace/1
  Demux1/1 -> RW1 saturation time counter/1(rate rpm)
  Mux3/1 -> Scope5/1
  Sum of Elements1/1 -> To Workspace2/1, Scope8/1  "Total power consumption of all theRW"
  Demux1/2 -> RW2 saturation time counter/1(rate rpm)
  RW3 saturation time counter/1(Out2) -> Mux2/3
  rad/s/1 -> Gain5/1, Angular Velocity Conversion2/1
  Gain/1 -> To Workspace12/1, Scope6/1  "Current consumption (mA)"
  RW4 saturation time counter/1(Out1) -> Mux2/4
  Demux2/3 -> Steady state Power consumption/3(RW3)
  Gain2/1 -> Abs1/1
  Gain5/1 -> Current gain for a 2mNm torque/1  "I_w"
  Demux2/4 -> Steady state Power consumption/4(RW4)
  RW1 saturation time counter/1(Out1) -> Mux2/1
  Angular Velocity Conversion2/1 -> Demux1/1, Demux2/1, To Workspace10/1  "rate rpm"
  Current gain for a 2mNm torque/1 -> Gain/1, Gain2/1, Gain7/1
  Steady state Power consumption/1(WP1) -> Mux3/1
  Steady state Power consumption/2(WP2) -> Mux3/2
  Steady state Power consumption/3(WP3) -> Mux3/3
  Demux2/1 -> Steady state Power consumption/1(RW1)
  Steady state Power consumption/4(WP4) -> Mux3/4

== system Control_v6_LQR_2020b_for_Monte_carlo/Attitude Controller/Reaction Wheels Speed Command ==
  " command (normal)" : Inport
  Command (B-dot) : Inport  Port=2
  B_dot mode (0/1) : Inport  Port=3
  If1 : If
  Merge : Merge
  Switch Case Action Subsystem3 : Subsystem  TreatAsAtomicUnit=on
  Switch Case Action Subsystem4 : Subsystem  TreatAsAtomicUnit=on
  output command : Outport  VectorParamsAs1DForOutWhenUnconnected=off
  wires:
  If1/2 -> Switch Case Action Subsystem4/Action
  If1/1 -> Switch Case Action Subsystem3/Action
  B_dot mode (0/1)/1 -> If1/1
  Command (B-dot)/1 -> Switch Case Action Subsystem3/1(In1)
  Merge/1 -> output command/1
  Switch Case Action Subsystem3/1(Out1) -> Merge/1
  Switch Case Action Subsystem4/1(Out1) -> Merge/2
  " command (normal)"/1 -> Switch Case Action Subsystem4/1(In1)

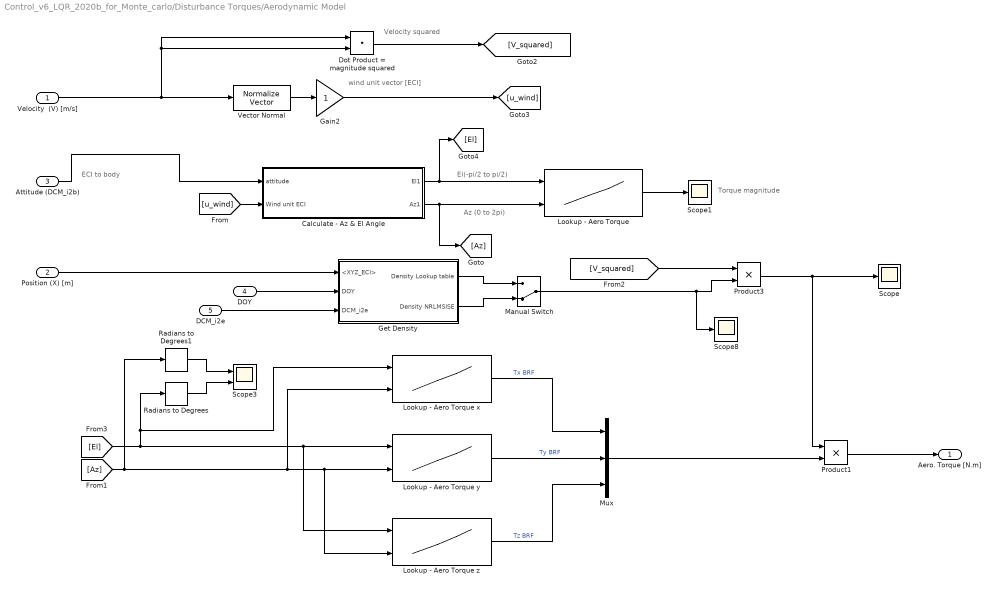
== system Control_v6_LQR_2020b_for_Monte_carlo/Disturbance Torques/Aerodynamic Model ==
  note: Az (0 to 2pi)
  note: wind unit vector [ECI]
  note: Torque magnitude
  note: ECI to body
  note: Velocity squared
  note: El(-pi/2 to pi/2)
  Velocity  (V) [m/s] : Inport
  Position (X) [m] : Inport  Port=2
  Attitude (DCM_i2b) : Inport  Port=3
  DOY : Inport  Port=4
  DCM_i2e : Inport  Port=5
  Calculate - Az & El Angle : Subsystem
  Dot Product = magnitude squared : DotProduct  InputSameDT=on  OutDataTypeStr=Inherit: Inherit via internal rule
  Gain2 : Gain
  Get Density : Subsystem
  Lookup - Aero Torque : Lookup2D  RowIndex=IonSataero.Az  ColumnIndex=IonSataero.El  Table=IonSataero.T
  Lookup - Aero Torque x : Lookup2D  RowIndex=IonSataero.Az  ColumnIndex=IonSataero.El  Table=IonSataero.Tx
  Lookup - Aero Torque y : Lookup2D  RowIndex=IonSataero.Az  ColumnIndex=IonSataero.El  Table=IonSataero.Ty
  Lookup - Aero Torque z : Lookup2D  RowIndex=IonSataero.Az  ColumnIndex=IonSataero.El  Table=IonSataero.Tz
  Manual Switch : ManualSwitch  CurrentSetting=0
  Mux : Mux  Inputs=3
  Product1 : Product  RndMeth=Zero
  Product3 : Product  RndMeth=Zero
  Radians to Degrees : simulink_extras/Transformations/Radians to Degrees
  Radians to Degrees1 : simulink_extras/Transformations/Radians to Degrees
  Scope : Scope
  Scope1 : Scope
  Scope3 : Scope  NumInputPorts=2
  Scope8 : Scope
  Vector Normal : vrlib/Utilities/Normalize Vector  maxzero=0
  Aero. Torque [N.m] : Outport
  wires:
  Dot Product = magnitude squared/1 -> [V_squared]
  Vector Normal/1 -> Gain2/1
  Gain2/1 -> [u_wind]
  Lookup - Aero Torque/1 -> Scope1/1
  Attitude (DCM_i2b)/1 -> Calculate - Az & El Angle/1(attitude)
  [V_squared] -> Product3/1
  Velocity  (V) [m/s]/1 -> Dot Product = magnitude squared/2, Dot Product = magnitude squared/1, Vector Normal/1
  Radians to Degrees1/1 -> Scope3/1
  Radians to Degrees/1 -> Scope3/2
  [u_wind] -> Calculate - Az & El Angle/2(Wind unit ECI)
  Calculate - Az & El Angle/2(Az1) -> [Az], Lookup - Aero Torque/2
  Calculate - Az & El Angle/1(El1) -> [El], Lookup - Aero Torque/1
  [El] -> Lookup - Aero Torque z/1, Lookup - Aero Torque y/1, Lookup - Aero Torque x/1, Radians to Degrees/1
  [Az] -> Radians to Degrees1/1, Lookup - Aero Torque z/2, Lookup - Aero Torque y/2, Lookup - Aero Torque x/2
  Lookup - Aero Torque y/1 -> Mux/2  "Ty BRF"
  Lookup - Aero Torque x/1 -> Mux/1  "Tx BRF"
  Lookup - Aero Torque z/1 -> Mux/3  "Tz BRF"
  Mux/1 -> Product1/2
  Product3/1 -> Product1/1, Scope/1
  Product1/1 -> Aero. Torque [N.m]/1
  Manual Switch/1 -> Scope8/1, Product3/2
  Position (X) [m]/1 -> Get Density/1(<XYZ_ECI>)
  DOY/1 -> Get Density/2(DOY)
  DCM_i2e/1 -> Get Density/3("DCM_i2e ")
  Get Density/2(Density NRLMSISE) -> Manual Switch/2
  Get Density/1(Density Lookup table) -> Manual Switch/1
